simulink model "W06_4_inner_loop"  (R2024b)
settings: Solver=FixedStepDiscrete  StartTime=0.0  StopTime=inf  FixedStep=0.05  RelTol=1e-3
libraries: ros2lib x5, slpidlib x1
settings Model: Creator=admin  LastModifiedBy=admin

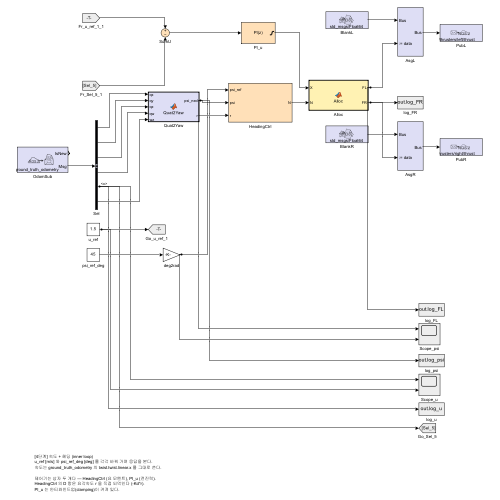
[thumbnail: Simulink's stored preview of the top-level diagram]
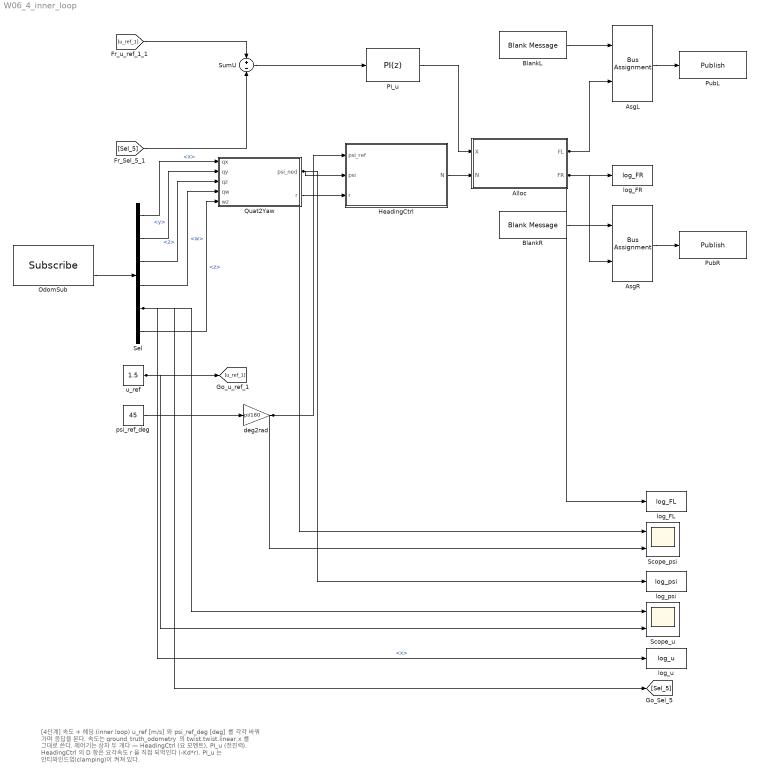
== system W06_4_inner_loop ==
  note: [4단계] 속도 + 헤딩 (inner loop)
      | u_ref [m/s] 와 psi_ref_deg [deg] 를 각각 바꿔 가며 응답을 본다.
      | 속도는 ground_truth_odometry 의 twist.twist.linear.x 를 그대로 쓴다.
      |
      | 제어기는 상자 두 개다 — HeadingCtrl (요 모멘트), PI_u (전진력).
      | HeadingCtrl 의 D 항은 요각속도 r 을 직접 되먹인다 (-Kd*r).
      | PI_u 는 안티와인드업(clamping)이 켜져 있다.
  Alloc : MATLAB Function  TreatAsAtomicUnit=on
  AsgL : BusAssignment  AssignedSignals=data
  AsgR : BusAssignment  AssignedSignals=data
  BlankL : ros2lib/Blank Message  messageClass=Message  entityType=std_msgs/Float64  messageType=std_msgs/Float64  SampleTime=0.05
  BlankR : ros2lib/Blank Message  messageClass=Message  entityType=std_msgs/Float64  messageType=std_msgs/Float64  SampleTime=0.05
  HeadingCtrl : Subsystem
  OdomSub : ros2lib/Subscribe  topicSource=Specify your own  topic=/wamv/sensors/position/ground_truth_odometry  messageType=nav_msgs/Odometry  sampleTime=0.05  QOSHistory=Keep last  QOSDepth=1  QOSReliability=Reliable  QOSDurability=Volatile  QOSDeadline=Inf  QOSLifespan=Inf  QOSLiveliness=Automatic  QOSLeaseDuration=Inf  QOSAvoidROSNamespaceConventions=off
  PI_u : slpidlib/PID Controller  Controller=PI  Form=Parallel  TimeDomain=Discrete-time  UseExternalTs=off  SampleTime=0.05  IntegratorMethod=Forward Euler  FilterMethod=Forward Euler  ControllerParametersSource=internal  P=300  I=40  UseKiTs=off  D=0  UseExternalDerivativeSource=off  N=100  UseFilter=on  TunerSelectOption=Transfer Function Based (PID Tuner App)  InitialConditionSource=internal  InitialConditionForIntegrator=0  InitialConditionForFilter=0  DifferentiatorICPrevScaledInput=0  ExternalReset=none  TrackingMode=off  Kt=1  LimitOutput=on  SatLimitsSource=internal  UpperSaturationLimit=500  LowerSaturationLimit=-500  LinearizeAsGain=off  AntiWindupMode=clamping  Kb=1  LimitIntegrator=off  UpperIntegratorSaturationLimit=inf  LowerIntegratorSaturationLimit=-inf  POutMin=[]  POutMax=[]  IOutMin=[]  IOutMax=[]  DOutMin=[]  DOutMax=[]  NOutMin=[]  NOutMax=[]  SumOutMin=[]  SumOutMax=[]  SaturationOutMin=[]  SaturationOutMax=[]  PParamMin=[]  PParamMax=[]  IParamMin=[]  IParamMax=[]  DParamMin=[]  DParamMax=[]  NParamMin=[]  NParamMax=[]  KbParamMin=[]  KbParamMax=[]  KtParamMin=[]  KtParamMax=[]  KbOutMin=[]  KbOutMax=[]  KtOutMin=[]  KtOutMax=[]  IntegratorOutMin=[]  IntegratorOutMax=[]  FilterOutMin=[]  FilterOutMax=[]  SumI1OutMin=[]  SumI1OutMax=[]  SumI2OutMin=[]  SumI2OutMax=[]  SumI3OutMin=[]  SumI3OutMax=[]  SumI4OutMin=[]  SumI4OutMax=[]  SumDOutMin=[]  SumDOutMax=[]  DifferentiatorOutMin=[]  DifferentiatorOutMax=[]  FilterDiffOutCoefMin=[]  FilterDiffOutCoefMax=[]  ReciprocalOutMin=[]  ReciprocalOutMax=[]  SumDenOutMin=[]  SumDenOutMax=[]  SumNumOutMin=[]  SumNumOutMax=[]  DivideOutMin=[]  DivideOutMax=[]  UdiffTsProdOutMin=[]  UdiffTsProdOutMax=[]  NTsProdOutMin=[]  NTsProdOutMax=[]  UintegralTsProdOutMin=[]  UintegralTsProdOutMax=[]  UngainTsProdOutMin=[]  UngainTsProdOutMax=[]  ClampingZeroOutDataTypeStr=Inherit: Inherit via back propagation  ClampingZeroOutMin=[]  ClampingZeroOutMax=[]  FilterDenConstantOutDataTypeStr=Inherit: Inherit via back propagation  FilterDenConstantOutMin=[]  FilterDenConstantOutMax=[]  PCopyOutDataTypeStr=Inherit: Inherit via back propagation  PCopyOutMin=[]  PCopyOutMax=[]  NCopyOutDataTypeStr=Inherit: Inherit via back propagation  NCopyOutMin=[]  NCopyOutMax=[]  IntegratorContinuousStateAttributes=''  IntegratorStateMustResolveToSignalObject=off  IntegratorRTWStateStorageClass=Auto  FilterContinuousStateAttributes=''  FilterStateMustResolveToSignalObject=off  FilterRTWStateStorageClass=Auto  ParallelPVariant=InternalParameters  IdealPVariant=Disabled  IVariant=InternalParameters  DVariant=Disabled  IntegratorVariant=Discrete  SatVariant=Enabled  AWVariant=DiscClampingParallel  PCopyVariant=Disabled  TRVariant=Disabled  FdbkBlocksVariant=Forward  IdealPFdbkVariant=Disabled  SatFdbkVariant=Disabled  DerivativeFilterVariant=Disabled  NVariant=Disabled  NCopyVariant=Disabled_SignalSpec  FilterICVariant=Disabled  IntegratorICVariant=InternalICs  ExternalResetVariant=Disabled  TRSumVariant=Passthrough  SumFdbkVariant=Disabled  SumVariant=Sum_PI  TsampFilterVariant=InternalTs  TsampNgainVariant=Passthrough  TsampIntegralVariant=Disabled_SignalSpec  ExternalSaturationOutDataTypeStr=Inherit: Same as second input  DerivativeSourceVariant=Disabled  PreIntVariant=InternalPreInt
      settings: LibrarySourceBlock=simulink/Discrete/Discrete PID Controller
  PubL : ros2lib/Publish  topicSource=Specify your own  topic=/wamv/thrusters/left/thrust  messageType=std_msgs/Float64  QOSHistory=Keep last  QOSDepth=1  QOSReliability=Reliable  QOSDurability=Volatile  QOSDeadline=Inf  QOSLifespan=Inf  QOSLiveliness=Automatic  QOSLeaseDuration=Inf  QOSAvoidROSNamespaceConventions=off
  PubR : ros2lib/Publish  topicSource=Specify your own  topic=/wamv/thrusters/right/thrust  messageType=std_msgs/Float64  QOSHistory=Keep last  QOSDepth=1  QOSReliability=Reliable  QOSDurability=Volatile  QOSDeadline=Inf  QOSLifespan=Inf  QOSLiveliness=Automatic  QOSLeaseDuration=Inf  QOSAvoidROSNamespaceConventions=off
  Quat2Yaw : MATLAB Function  TreatAsAtomicUnit=on
  Scope_psi : Scope  NumInputPorts=2
  Scope_u : Scope  NumInputPorts=2
  Sel : BusSelector  OutputSignals=pose.pose.orientation.x,pose.pose.orientation.y,pose.pose.orientation.z,pose.pose.orientation.w,twist.twist.linear.x,twist.twist.angular.z
  SumU : Sum  Inputs=+-
  deg2rad : Gain  Gain=pi/180
  log_FL : ToWorkspace  VariableName=log_FL  SaveFormat=Timeseries  SampleTime=0.05
  log_FR : ToWorkspace  VariableName=log_FR  SaveFormat=Timeseries  SampleTime=0.05
  log_psi : ToWorkspace  VariableName=log_psi  SaveFormat=Timeseries  SampleTime=0.05
  log_u : ToWorkspace  VariableName=log_u  SaveFormat=Timeseries  SampleTime=0.05
  psi_ref_deg : Constant  Value=45
  u_ref : Constant  Value=1.5
  wires:
  Sel/4 -> Quat2Yaw/4(qw)  "<w>"
  OdomSub/2 -> Sel/1
  [u_ref_1] -> SumU/1
  Sel/1 -> Quat2Yaw/1(qx)  "<x>"
  [Sel_5] -> SumU/2
  Sel/2 -> Quat2Yaw/2(qy)  "<y>"
  Sel/3 -> Quat2Yaw/3(qz)  "<z>"
  Sel/6 -> Quat2Yaw/5(wz)  "<z>"
  u_ref/1 -> [u_ref_1], Scope_u/2
  psi_ref_deg/1 -> deg2rad/1
  HeadingCtrl/1(N) -> Alloc/2(N)
  SumU/1 -> PI_u/1
  Quat2Yaw/2(r) -> HeadingCtrl/3(r)
  Quat2Yaw/1(psi_ned) -> HeadingCtrl/2(psi), Scope_psi/1, log_psi/1
  deg2rad/1 -> HeadingCtrl/1(psi_ref), Scope_psi/2
  PI_u/1 -> Alloc/1(X)
  BlankL/1 -> AsgL/1
  Alloc/1(FL) -> AsgL/2, log_FL/1
  Alloc/2(FR) -> AsgR/2, log_FR/1
  BlankR/1 -> AsgR/1
  AsgL/1 -> PubL/1
  AsgR/1 -> PubR/1
  Sel/5 -> log_u/1, [Sel_5], Scope_u/1  "<x>"

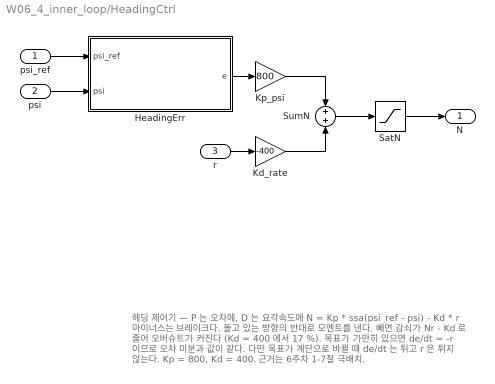
== system W06_4_inner_loop/HeadingCtrl ==
  note: 헤딩 제어기 — P 는 오차에, D 는 요각속도에
      |
      |     N = Kp * ssa(psi_ref - psi)  -  Kd * r
      |
      | 마이너스는 브레이크다. 돌고 있는 방향의 반대로 모멘트를 낸다.
      | 빼면 감쇠가 Nr - Kd 로 줄어 오버슈트가 커진다 (Kd = 400 에서 17 %).
      |
      | 목표가 가만히 있으면 de/dt = -r 이므로 오차 미분과 값이 같다.
      | 다만 목표가 계단으로 바뀔 때 de/dt 는 튀고 r 은 튀지 않는다.
      |
      | Kp = 800, Kd = 400.  근거는 6주차 1-7절 극배치.
  psi_ref : Inport
  psi : Inport  Port=2
  r : Inport  Port=3
  HeadingErr : MATLAB Function  TreatAsAtomicUnit=on
  Kd_rate : Gain  Gain=-400
  Kp_psi : Gain  Gain=800
  SatN : Saturate  UpperLimit=500  LowerLimit=-500
  SumN : Sum
  N : Outport
  wires:
  Kd_rate/1 -> SumN/2
  psi_ref/1 -> HeadingErr/1(psi_ref)
  Kp_psi/1 -> SumN/1
  psi/1 -> HeadingErr/2(psi)
  HeadingErr/1(e) -> Kp_psi/1
  r/1 -> Kd_rate/1
  SumN/1 -> SatN/1
  SatN/1 -> N/1

== matlab function W06_4_inner_loop/HeadingCtrl/HeadingErr ==
  data: psi_ref input; e output; psi input
function e = HeadingErr(psi_ref, psi)
%#codegen
% Shortest signed angle, wrapped to [-pi, pi]
d = psi_ref - psi;
e = atan2(sin(d), cos(d));

== matlab function W06_4_inner_loop/Quat2Yaw ==
  data: qx input; psi_ned output; qy input; qz input; qw input; wz input; r output
function [psi_ned, r] = Quat2Yaw(qx, qy, qz, qw, wz)
%#codegen
% ROS quaternion (ENU body) -> NED heading [rad] and yaw rate [rad/s]
yaw_enu = atan2(2*(qw*qz + qx*qy), 1 - 2*(qy*qy + qz*qz));
psi = pi/2 - yaw_enu;
psi_ned = atan2(sin(psi), cos(psi));   % wrap to [-pi, pi]

% psi_ned = pi/2 - yaw_enu  ->  d(psi_ned)/dt = -d(yaw_enu)/dt.
% ENU is z-up and NED is z-down, so the turn direction flips.
r = -wz;

== matlab function W06_4_inner_loop/Alloc ==
  data: X input; FL output; N input; FR output
function [FL, FR] = Alloc(X, N)
%#codegen
% Differential thrust allocation for the 2-thruster WAM-V
%   X : surge force  [N]
%   N : yaw moment   [N*m], positive turns to starboard
B_half = 1.027135;      % half distance between thrusters [m]
Fmax   = 250;           % thrust limit per thruster [N]
FL = X/2 + N/(2*B_half);
FR = X/2 - N/(2*B_half);
FL = max(min(FL, Fmax), -Fmax);
FR = max(min(FR, Fmax), -Fmax);
